simulink model "nex"  (R2020b)
settings: Solver=VariableStepAuto  StartTime=0.0  StopTime=1000.0  RelTol=1e-3
libraries: simulink x1
settings Model: Creator=morro  LastModifiedBy=morro

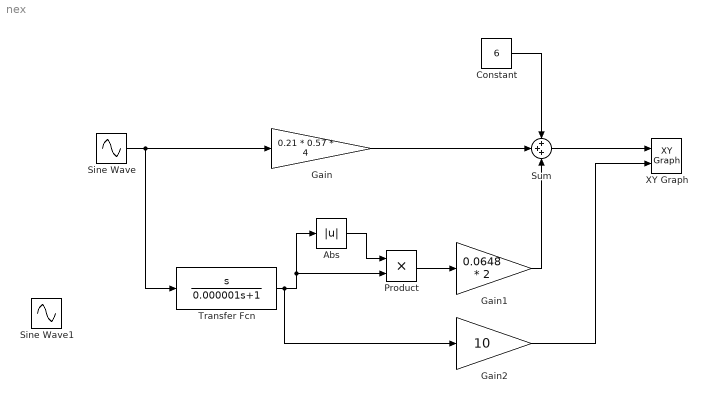
== system nex ==
  Abs : Abs
  Constant : Constant  Value=6
  Gain : Gain  Gain=0.21 * 0.57 * 4
  Gain1 : Gain  Gain=0.0648 * 2
  Gain2 : Gain  Gain=10
  Product : Product
  Sine Wave : Sin  Amplitude=3.5  Frequency=0.57  SampleTime=0
  Sine Wave1 : Sin  Amplitude=3.5  Frequency=0.57  Phase=0.5  SampleTime=0
  Sum : Sum  Inputs=+++
  Transfer Fcn : TransferFcn  Numerator=[1 0]  Denominator=[0.000001 1]
  XY Graph : simulink/Sinks/XY Graph  xmin=4  xmax=8  ymin=-25  ymax=25  st=-1
  wires:
  Sine Wave/1 -> Transfer Fcn/1, Gain/1
  Sum/1 -> XY Graph/1
  Product/1 -> Gain1/1
  Abs/1 -> Product/1
  Gain/1 -> Sum/2
  Gain1/1 -> Sum/3
  Gain2/1 -> XY Graph/2
  Constant/1 -> Sum/1
  Transfer Fcn/1 -> Gain2/1, Product/2, Abs/1
